simulink model "gtcs_mcb_v0"  (R2022a)
settings: Solver=VariableStepAuto  StartTime=0.0  StopTime=10.0  RelTol=1e-3
undefined symbols (not defined in the file or in its folder): inverter, pmsm, Ts_motor, Ts_simulink
libraries: mcbcontrolslib x2, autolibpmsmexterior x2, mcbplantlib x1
settings Model: Creator=yusuf.ogut  LastModifiedBy=yusuf.ogut

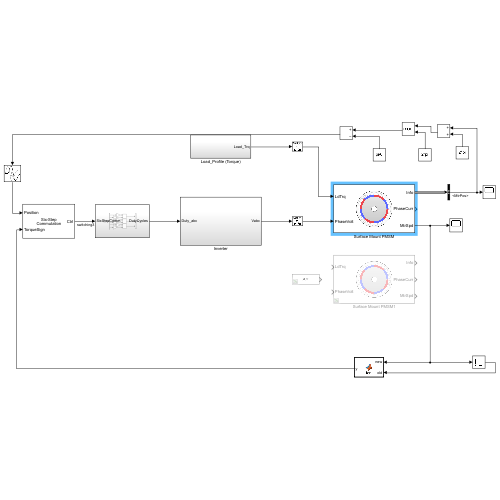
[thumbnail: Simulink's stored preview of the top-level diagram]
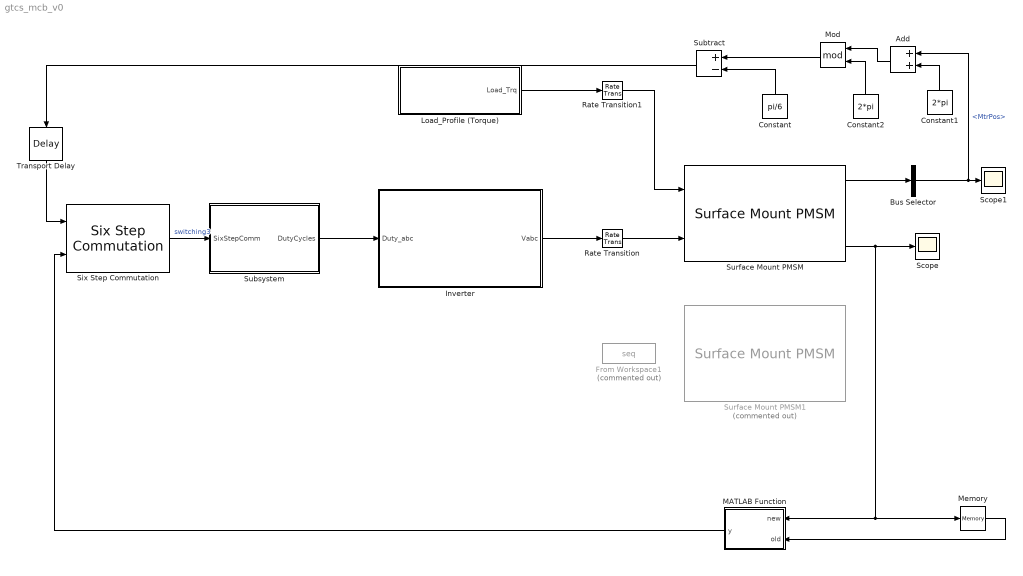
== system gtcs_mcb_v0 ==
  Add : Sum
  Bus Selector : BusSelector  OutputSignals=MtrPos
  Constant : Constant  Value=pi/6
  Constant1 : Constant  Value=2*pi
  Constant2 : Constant  Value=2*pi
  From Workspace1 : FromWorkspace  Commented=on  VariableName=seq
  Inverter : Subsystem
  Load_Profile (Torque) : Subsystem
  MATLAB Function : MATLAB Function  TreatAsAtomicUnit=on
  Memory : Memory
  Mod : Math  Operator=mod
  Rate Transition : RateTransition  Deterministic=off  OutPortSampleTime=Ts_motor
  Rate Transition1 : RateTransition  Deterministic=off  OutPortSampleTime=Ts_motor
  Scope : Scope
  Scope1 : Scope
  Six Step Commutation : mcbcontrolslib/Six Step Commutation  InputType=Position  PositionUnit=Radians  CommutationMode=120 deg  SequencePos=[5,4,6,2,3,1]  EnableCustomSwitching=off  CommutationSeqPos=[0 0 1 0 0 1;0 1 1 0 0 0;0 1 0 0 1 0;0 0 0 1 1 0;1 0 0 1 0 0;1 0 0 0 0 1]  CommutationSeqNeg="[0  1  1  0  0  0;0  1  0  0  1  0;0  0  0  1  1  0;1  0  0  1  0  0;1  0  0  0  0  1;0  0  1  0  0  1;]"
      settings: SourceProductBaseCode=MT
  Subsystem : Subsystem
  Subtract : Sum  Inputs=+-
  Surface Mount PMSM : autolibpmsmexterior/Surface Mount PMSM  port_config=Torque  sim_type=Discrete  Ts=Ts_motor  P=2  Rs=0.045  Ldq_=15e-06  KConstText=Torque constant (Kt):  lambda_pm=pmsm.FluxPM  Ke=159.9771  Kt=0.040  mechanical=[pmsm.J, pmsm.B, 0]  idq0=[0 0]  theta_init=0  omega_init=0  KConst=0.040  lambda_pm_calc=0.013333  RefBlkName='autolibpmsmexterior/Surface Mount PMSM'  aMode=5  Ldq="[0.0006      0.0006]"
      settings: SourceProductBaseCode=PW,DR,MT,VE
  Surface Mount PMSM1 : autolibpmsmexterior/Surface Mount PMSM  Commented=on  port_config=Torque  sim_type=Discrete  Ts=Ts_motor  P=pmsm.p  Rs=pmsm.Rs + inverter.R_board  Ldq_=pmsm.Ld  KConstText=Permanent flux linkage constant (lambda_pm):  lambda_pm=pmsm.FluxPM  Ke=159.9771  Kt=1.323  mechanical=[pmsm.J, pmsm.B, 0]  idq0=[0 0]  theta_init=0  omega_init=0  KConst=pmsm.FluxPM  lambda_pm_calc=pmsm.FluxPM  RefBlkName='autolibpmsmexterior/Surface Mount PMSM'  aMode=5  Ldq="[0.0006      0.0006]"
      settings: SourceProductBaseCode=PW,DR,MT,VE
  Transport Delay : TransportDelay  DelayTime=0.5
  wires:
  Load_Profile (Torque)/1(Load_Trq) -> Rate Transition1/1
  Inverter/1(Vabc) -> Rate Transition/1
  Rate Transition/1 -> Surface Mount PMSM/2
  Surface Mount PMSM/3 -> MATLAB Function/1(new), Memory/1, Scope/1
  Surface Mount PMSM/1 -> Bus Selector/1
  Bus Selector/1 -> Add/1, Scope1/1  "<MtrPos>"
  MATLAB Function/1(y) -> Six Step Commutation/2
  Six Step Commutation/1 -> Subsystem/1(SixStepComm)  "switching3"
  Constant/1 -> Subtract/2
  Subtract/1 -> Transport Delay/1
  Memory/1 -> MATLAB Function/2(old)
  Transport Delay/1 -> Six Step Commutation/1
  Subsystem/1(DutyCycles) -> Inverter/1(Duty_abc)
  Constant1/1 -> Add/2
  Add/1 -> Mod/1
  Constant2/1 -> Mod/2
  Mod/1 -> Subtract/1
  Rate Transition1/1 -> Surface Mount PMSM/1

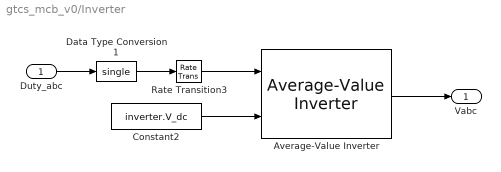
== system gtcs_mcb_v0/Inverter ==
  Duty_abc : Inport
  Average-Value Inverter : mcbplantlib/Average-Value Inverter
  Constant2 : Constant  Value=inverter.V_dc  OutDataTypeStr=single  SampleTime=-1
  Data Type Conversion1 : DataTypeConversion  OutDataTypeStr=single  RndMeth=Simplest  SaturateOnIntegerOverflow=off
  Rate Transition3 : RateTransition  Deterministic=off  OutPortSampleTime=Ts_inverter
  Vabc : Outport  VectorParamsAs1DForOutWhenUnconnected=off
  wires:
  Average-Value Inverter/1 -> Vabc/1
  Constant2/1 -> Average-Value Inverter/2
  Rate Transition3/1 -> Average-Value Inverter/1
  Duty_abc/1 -> Data Type Conversion1/1
  Data Type Conversion1/1 -> Rate Transition3/1

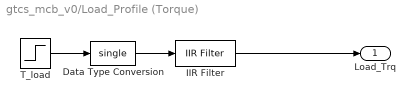
== system gtcs_mcb_v0/Load_Profile (Torque) ==
  Data Type Conversion : DataTypeConversion  OutDataTypeStr=single  SaturateOnIntegerOverflow=off  RndMeth=Floor
  IIR Filter : mcbcontrolslib/IIR Filter  VariantControl=Low Pass Filter  VariantSelect=Low-pass  Filter_constant=0.01  advancedSettings=off  Ts=50e-6  cutOff_freq=32.1525
      settings: SourceProductBaseCode=MT
  T_load : Step  Time=5  Before=0.05*pmsm.T_rated  After=0.5*pmsm.T_rated  SampleTime=Ts_simulink
  Load_Trq : Outport  VectorParamsAs1DForOutWhenUnconnected=off
  wires:
  IIR Filter/1 -> Load_Trq/1
  Data Type Conversion/1 -> IIR Filter/1
  T_load/1 -> Data Type Conversion/1

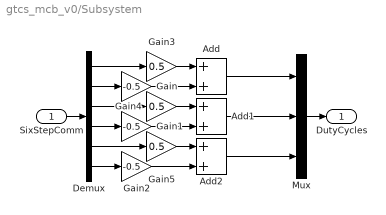
== system gtcs_mcb_v0/Subsystem ==
  SixStepComm : Inport
  Add : Sum
  Add1 : Sum
  Add2 : Sum
  Demux : Demux  Outputs=6
  Gain : Gain  Gain=-0.5
  Gain1 : Gain  Gain=-0.5
  Gain2 : Gain  Gain=-0.5
  Gain3 : Gain  Gain=0.5
  Gain4 : Gain  Gain=0.5
  Gain5 : Gain  Gain=0.5
  Mux : Mux  Inputs=3
  DutyCycles : Outport
  wires:
  Add1/1 -> Mux/2
  Demux/3 -> Gain4/1
  Demux/5 -> Gain5/1
  Demux/4 -> Gain1/1
  SixStepComm/1 -> Demux/1
  Demux/1 -> Gain3/1
  Gain2/1 -> Add2/2
  Add2/1 -> Mux/3
  Demux/2 -> Gain/1
  Gain/1 -> Add/2
  Gain1/1 -> Add1/2
  Mux/1 -> DutyCycles/1
  Add/1 -> Mux/1
  Demux/6 -> Gain2/1
  Gain3/1 -> Add/1
  Gain4/1 -> Add1/1
  Gain5/1 -> Add2/1

== matlab function gtcs_mcb_v0/MATLAB Function ==
  data: new input; y output; old input
function y = fcn(new, old)
    y = 1;
    if new<old
        y = -1;
    end
end
